simulink subsystem "EKF"  (R2021a)
settings: Solver=VariableStepAuto  StartTime=0.0  StopTime=10.0  RelTol=1e-3
settings Model: Creator=Laura  LastModifiedBy=Laura

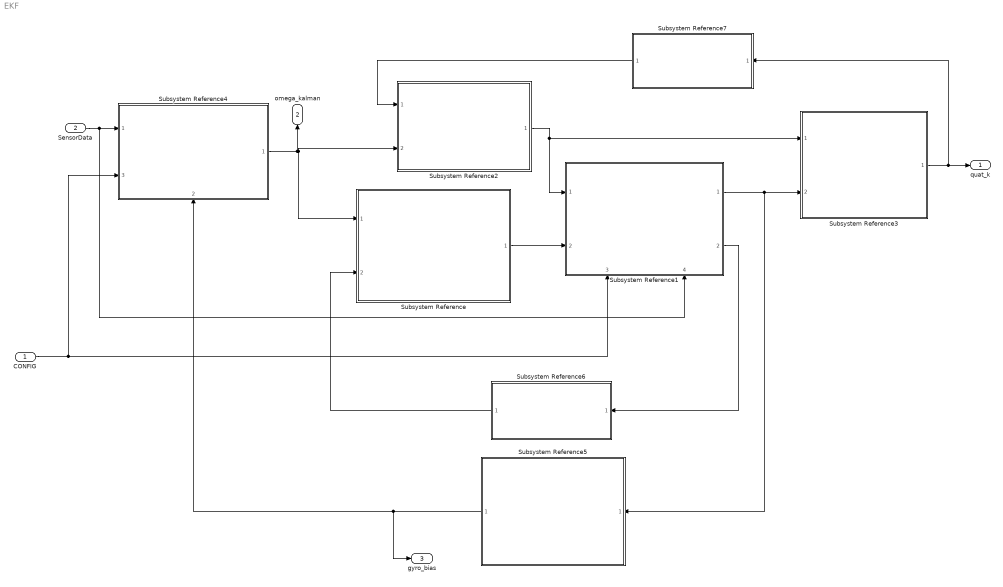
== system EKF ==
  CONFIG : Inport
  SensorData : Inport  Port=2
  Subsystem Reference : Subsystem  ReferencedSubsystem=EKF_prediction
  Subsystem Reference1 : Subsystem  ReferencedSubsystem=EKF_correction
      settings: PortSchema="{\"entries\":[{\"content\":{\"sides\":[{\"content\":{\"connectorIds\":[\"In1\",\"In2\"]},\"type\":\"ConnectorPlacement.EquallySpacedRectSide\",\"uuid\":\"455e34a3-a605-4fd6-a99e-9e182f6df0f1\"},{\"content\":{\"connectorIds\":[\"Out1\",\"Out2\"],\"side\":\"RIGHT\"},\"type\":\"ConnectorPlacement.EquallySpacedRectSide\",\"uuid\":\"a616d48d-08ce-4ae0-9e16-9241222a1826\"},{\"content\":{\"connectorIds\":[],\"side\":\"TOP\"},\"type\":\"ConnectorPlacement.EquallySpacedRectSide\",\"uuid\":\"a620cff5-5999-407b-8f43-1d9fdb5ea25d\"},{\"content\":{\"connectorIds\":[\"In3\",\"In4\"],\"side\":\"BOTTOM\"},\"type\":\"ConnectorPlacement.EquallySpacedRectSide\",\"uuid\":\"b464cb54-5a80-441b-98f4-0f455ac8c87f\"}]},\"type\":\"ConnectorPlacement.EquallySpacedConnector\",\"uuid\":\"2aa0ef96-04e1-4ff7-bd11-918b03e6d51b\"}],\"packageUris\":[\"http://schema.mathworks.com/mf0/Connector/R2020b\"],\"version\":\"1.0\"}"
  Subsystem Reference2 : Subsystem  ReferencedSubsystem=EKF_GyroIntegrator
  Subsystem Reference3 : Subsystem  ReferencedSubsystem=QuaternionUpdate
  Subsystem Reference4 : Subsystem  ReferencedSubsystem=CorrectAngVelocity
      settings: PortSchema="{\"entries\":[{\"content\":{\"sides\":[{\"content\":{\"connectorIds\":[\"In1\",\"In3\"]},\"type\":\"ConnectorPlacement.EquallySpacedRectSide\",\"uuid\":\"80b60f82-5988-494c-9d80-c4cf3c6744a7\"},{\"content\":{\"connectorIds\":[\"Out1\"],\"side\":\"RIGHT\"},\"type\":\"ConnectorPlacement.EquallySpacedRectSide\",\"uuid\":\"a3aaaeb4-4e89-4e97-9e0c-438e158dfcd8\"},{\"content\":{\"connectorIds\":[],\"side\":\"TOP\"},\"type\":\"ConnectorPlacement.EquallySpacedRectSide\",\"uuid\":\"44532c6d-b294-42a4-bd08-55822350bfda\"},{\"content\":{\"connectorIds\":[\"In2\"],\"side\":\"BOTTOM\"},\"type\":\"ConnectorPlacement.EquallySpacedRectSide\",\"uuid\":\"cad00d1c-3f8e-45a6-9486-3336315ed6df\"}]},\"type\":\"ConnectorPlacement.EquallySpacedConnector\",\"uuid\":\"f7d204d0-4a0a-460c-a502-497d13172aee\"}],\"packageUris\":[\"http://schema.mathworks.com/mf0/Connector/R2020b\"],\"version\":\"1.0\"}"
  Subsystem Reference5 : Subsystem  ReferencedSubsystem=BiasUpdate
  Subsystem Reference6 : Subsystem  ReferencedSubsystem=StateCovarianceInit
  Subsystem Reference7 : Subsystem  ReferencedSubsystem=QuaternionInit
  quat_k : Outport  LockScale=on
  omega_kalman : Outport  Port=2
  gyro_bias : Outport  Port=3
  wires:
  Subsystem Reference/1 -> Subsystem Reference1/2
  Subsystem Reference3/1 -> quat_k/1, Subsystem Reference7/1
  CONFIG/1 -> Subsystem Reference1/3, Subsystem Reference4/3
  SensorData/1 -> Subsystem Reference4/1, Subsystem Reference1/4
  Subsystem Reference4/1 -> omega_kalman/1, Subsystem Reference/1, Subsystem Reference2/2
  Subsystem Reference1/2 -> Subsystem Reference6/1
  Subsystem Reference6/1 -> Subsystem Reference/2
  Subsystem Reference5/1 -> Subsystem Reference4/2, gyro_bias/1
  Subsystem Reference1/1 -> Subsystem Reference3/2, Subsystem Reference5/1
  Subsystem Reference7/1 -> Subsystem Reference2/1
  Subsystem Reference2/1 -> Subsystem Reference1/1, Subsystem Reference3/1
